simulink model "TST_SyC_Main"  (R2016b)
settings: Solver=FixedStepDiscrete  StartTime=0.0  StopTime=simTime  FixedStep=sampleTime  RelTol=1e-3
values from neighbouring files (symbols this model uses):
  testCase = 1    [initTST_SyC_Main_001.m]
libraries: simulink x2, UnitTest_Lib x2
settings Model: Creator=liangyunbo  LastModifiedBy=liangyunbo
settings DebuggingCC: SignalRangeChecking=error

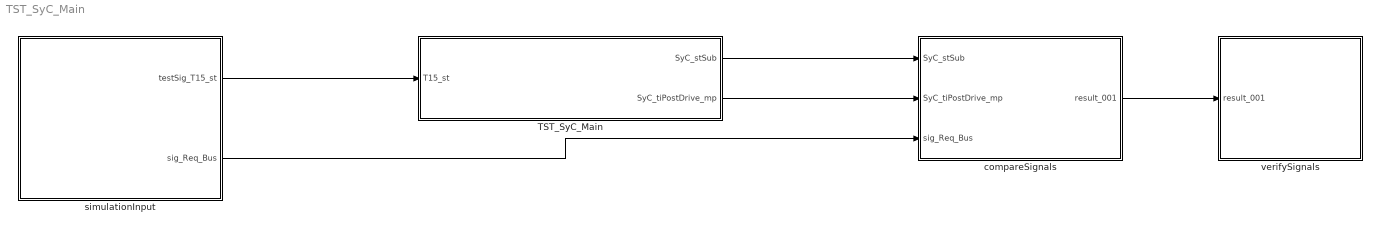
== system TST_SyC_Main ==
  TST_SyC_Main : Subsystem
  compareSignals : Subsystem
  simulationInput : Subsystem
  verifySignals : Subsystem
  wires:
  simulationInput/1(testSig_T15_st) -> TST_SyC_Main/1(T15_st)
  TST_SyC_Main/1(SyC_stSub) -> compareSignals/1(SyC_stSub)
  TST_SyC_Main/2(SyC_tiPostDrive_mp) -> compareSignals/2(SyC_tiPostDrive_mp)
  simulationInput/2(sig_Req_Bus) -> compareSignals/3(sig_Req_Bus)
  compareSignals/1(result_001) -> verifySignals/1(result_001)

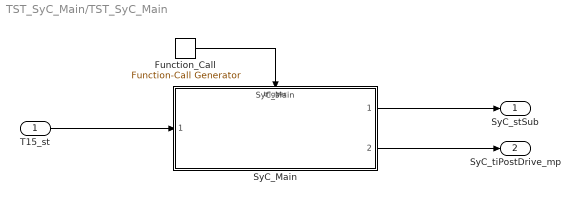
== system TST_SyC_Main/TST_SyC_Main ==
  T15_st : Inport
  Function_Call : simulink/Ports & Subsystems/Function-Call Generator  sample_time=sampleTime  numberOfIterations=1
  SyC_Main : ModelReference  ModelNameDialog=SyC_Main  SimulationMode=Normal  ModelReferenceVersion=1.10  TriggerPortName=function  TriggerPortTriggerType=function-call  TriggerPortStatesWhenEnabling=held
  SyC_stSub : Outport
  SyC_tiPostDrive_mp : Outport  Port=2
  wires:
  Function_Call/1 -> SyC_Main/Trigger
  T15_st/1 -> SyC_Main/1
  SyC_Main/1 -> SyC_stSub/1
  SyC_Main/2 -> SyC_tiPostDrive_mp/1

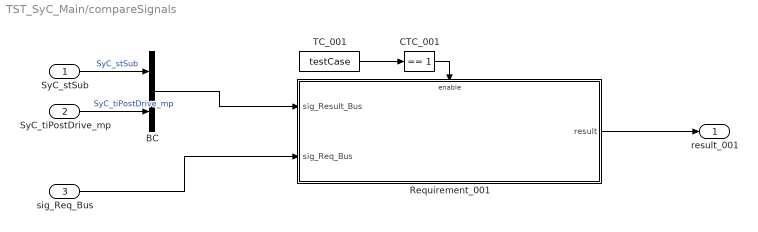
== system TST_SyC_Main/compareSignals ==
  SyC_stSub : Inport
  SyC_tiPostDrive_mp : Inport  Port=2
  sig_Req_Bus : Inport  Port=3
  BC : BusCreator  Inputs=2
  CTC_001 : simulink/Logic and Bit Operations/Compare To Constant  relop===  const=1  OutDataTypeStr=boolean
  Requirement_001 : Subsystem
  TC_001 : Constant  Value=testCase
  result_001 : Outport
  wires:
  SyC_stSub/1 -> BC/1  "SyC_stSub"
  SyC_tiPostDrive_mp/1 -> BC/2  "SyC_tiPostDrive_mp"
  TC_001/1 -> CTC_001/1
  CTC_001/1 -> Requirement_001/Enable
  sig_Req_Bus/1 -> Requirement_001/2(sig_Req_Bus)
  BC/1 -> Requirement_001/1(sig_Result_Bus)
  Requirement_001/1(result) -> result_001/1

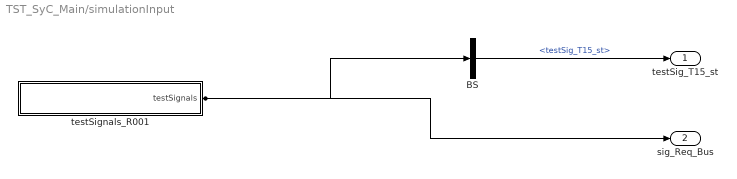
== system TST_SyC_Main/simulationInput ==
  BS : BusSelector  OutputSignals=testSig_T15_st
  testSignals_R001 : Subsystem
  testSig_T15_st : Outport
  sig_Req_Bus : Outport  Port=2
  wires:
  BS/1 -> testSig_T15_st/1  "<testSig_T15_st>"
  testSignals_R001/1(testSignals) -> BS/1, sig_Req_Bus/1

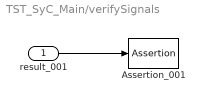
== system TST_SyC_Main/verifySignals ==
  result_001 : Inport
  Assertion_001 : Assertion  Enabled=off
  wires:
  result_001/1 -> Assertion_001/1

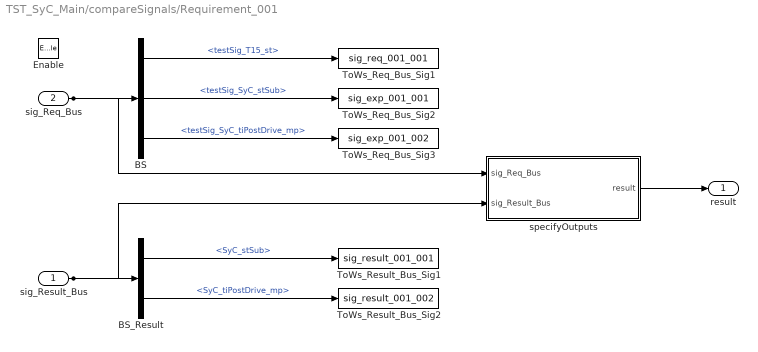
== system TST_SyC_Main/compareSignals/Requirement_001 ==
  sig_Result_Bus : Inport
  sig_Req_Bus : Inport  Port=2
  Enable : EnablePort
  BS : BusSelector  OutputSignals=testSig_T15_st,testSig_SyC_stSub,testSig_SyC_tiPostDrive_mp
  BS_Result : BusSelector  OutputSignals=SyC_stSub,SyC_tiPostDrive_mp
  ToWs_Req_Bus_Sig1 : ToWorkspace  VariableName=sig_req_001_001  SaveFormat=Structure With Time
  ToWs_Req_Bus_Sig2 : ToWorkspace  VariableName=sig_exp_001_001  SaveFormat=Structure With Time
  ToWs_Req_Bus_Sig3 : ToWorkspace  VariableName=sig_exp_001_002  SaveFormat=Structure With Time
  ToWs_Result_Bus_Sig1 : ToWorkspace  VariableName=sig_result_001_001  SaveFormat=Structure With Time
  ToWs_Result_Bus_Sig2 : ToWorkspace  VariableName=sig_result_001_002  SaveFormat=Structure With Time
  specifyOutputs : Subsystem
  result : Outport
  wires:
  sig_Req_Bus/1 -> BS/1, specifyOutputs/1(sig_Req_Bus)
  BS/1 -> ToWs_Req_Bus_Sig1/1  "<testSig_T15_st>"
  BS/2 -> ToWs_Req_Bus_Sig2/1  "<testSig_SyC_stSub>"
  BS/3 -> ToWs_Req_Bus_Sig3/1  "<testSig_SyC_tiPostDrive_mp>"
  sig_Result_Bus/1 -> BS_Result/1, specifyOutputs/2(sig_Result_Bus)
  BS_Result/1 -> ToWs_Result_Bus_Sig1/1  "<SyC_stSub>"
  BS_Result/2 -> ToWs_Result_Bus_Sig2/1  "<SyC_tiPostDrive_mp>"
  specifyOutputs/1(result) -> result/1

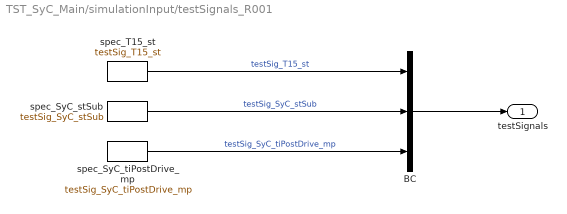
== system TST_SyC_Main/simulationInput/testSignals_R001 ==
  BC : BusCreator  Inputs=3
  spec_SyC_stSub : FromWorkspace  VariableName=testSig_SyC_stSub  Interpolate=off  OutputAfterFinalValue=Holding final value
  spec_SyC_tiPostDrive_mp : FromWorkspace  VariableName=testSig_SyC_tiPostDrive_mp  Interpolate=off  OutputAfterFinalValue=Holding final value
  spec_T15_st : FromWorkspace  VariableName=testSig_T15_st  Interpolate=off  OutputAfterFinalValue=Holding final value
  testSignals : Outport
  wires:
  BC/1 -> testSignals/1
  spec_T15_st/1 -> BC/1  "testSig_T15_st"
  spec_SyC_stSub/1 -> BC/2  "testSig_SyC_stSub"
  spec_SyC_tiPostDrive_mp/1 -> BC/3  "testSig_SyC_tiPostDrive_mp"

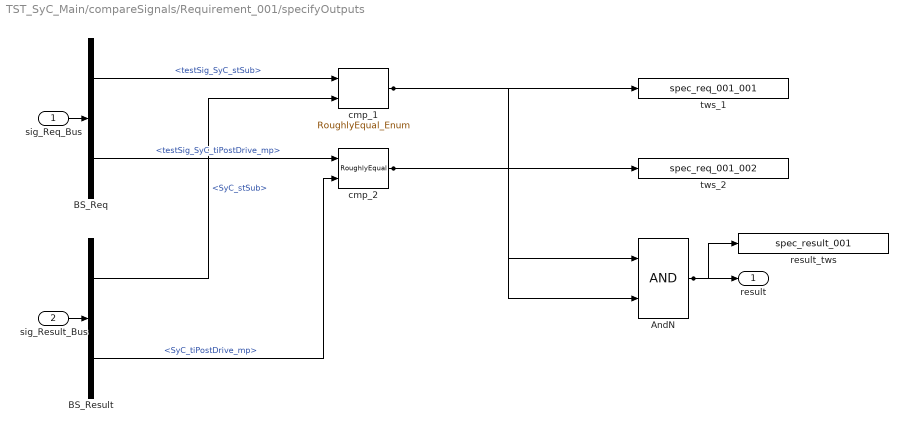
== system TST_SyC_Main/compareSignals/Requirement_001/specifyOutputs ==
  sig_Req_Bus : Inport
  sig_Result_Bus : Inport  Port=2
  AndN : Logic
  BS_Req : BusSelector  OutputSignals=testSig_SyC_stSub,testSig_SyC_tiPostDrive_mp
  BS_Result : BusSelector  OutputSignals=SyC_stSub,SyC_tiPostDrive_mp
  cmp_1 : UnitTest_Lib/RoughlyEqual_Enum  slope=0.1
  cmp_2 : UnitTest_Lib/RoughlyEqual  slope=0.1
  result_tws : ToWorkspace  VariableName=spec_result_001
  tws_1 : ToWorkspace  VariableName=spec_req_001_001
  tws_2 : ToWorkspace  VariableName=spec_req_001_002
  result : Outport
  wires:
  sig_Req_Bus/1 -> BS_Req/1
  sig_Result_Bus/1 -> BS_Result/1
  AndN/1 -> result/1, result_tws/1
  BS_Req/1 -> cmp_1/1  "<testSig_SyC_stSub>"
  BS_Result/1 -> cmp_1/2  "<SyC_stSub>"
  cmp_1/1 -> tws_1/1, AndN/1
  BS_Req/2 -> cmp_2/1  "<testSig_SyC_tiPostDrive_mp>"
  BS_Result/2 -> cmp_2/2  "<SyC_tiPostDrive_mp>"
  cmp_2/1 -> tws_2/1, AndN/2
